simulink model "nmpcSim"  (R2024b)
settings: Solver=FixedStepAuto  StartTime=0.0  StopTime=150  RelTol=1e-3
values from neighbouring files (symbols this model uses):
  C = zeros(4,6)    [outputFcnJacobian.m]
undefined symbols (not defined in the file or in its folder): A, B, Dx, Dy, p_msg, R_gps, R_imu, R_mag, Ts, Ts_gps, Ts_imu, Ts_mag, wps, x_ref, x_ref2, y_ref, y_ref2
libraries: simulink x4, sharedTrackingLibrary x1, dspstat3 x1, mpclib x1
settings Model: Creator=mpilo  LastModifiedBy=mpilo

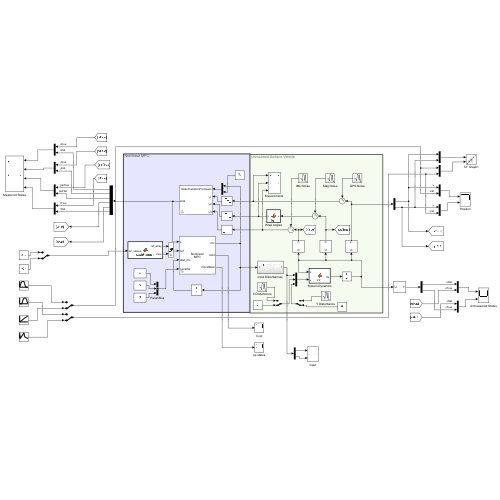
[thumbnail: Simulink's stored preview of the top-level diagram]
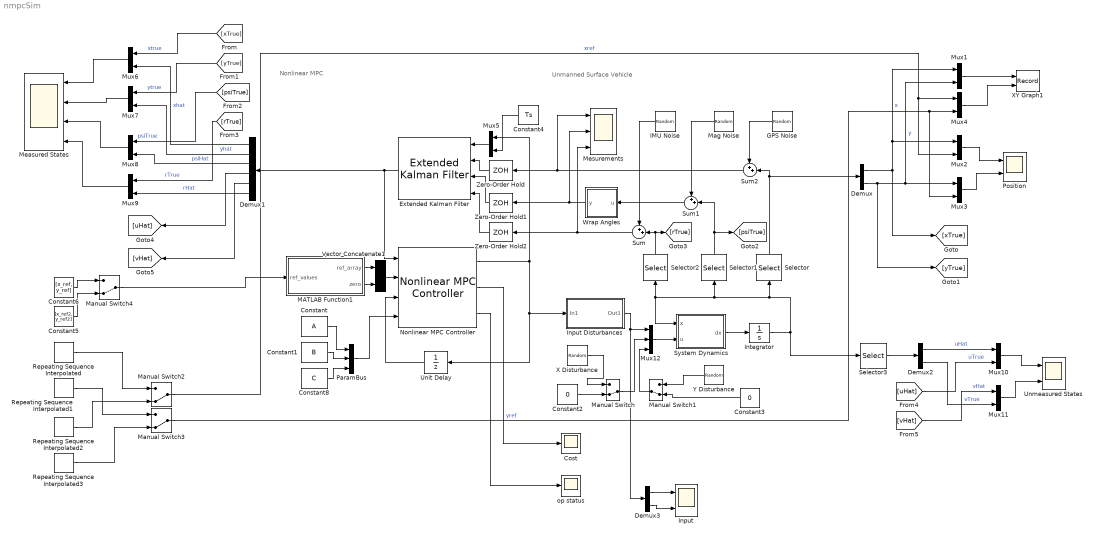
== system nmpcSim ==
  note: Nonlinear MPC
  note: Unmanned Surface Vehicle
  Constant : Constant  Value=A
  Constant1 : Constant  Value=B
  Constant2 : Constant  Value=0
  Constant3 : Constant  Value=0
  Constant4 : Constant  Value=Ts
  Constant5 : Constant  Value=[x_ref2, y_ref2]
  Constant6 : Constant  Value=[x_ref, y_ref]
  Constant8 : Constant  Value=C
  Cost : Scope
  Demux : Demux  Outputs=2
  Demux1 : Demux  Outputs=6
  Demux2 : Demux  Outputs=2
  Demux3 : Demux  Outputs=2
  Extended Kalman Filter : sharedTrackingLibrary/Extended Kalman Filter  StateTransitionFcn=stateTransitionFcnDT  HasStateTransitionJacobianFcn=off  StateTransitionJacobianFcn=stateTransitionFcnJacobian  HasAdditiveProcessNoise=Additive  ProcessNoise=Q  HasTimeVaryingProcessNoise=off  HasStateTransitionFcnExtraArgument=1  InitialState=x0  InitialStateCovariance=P_0  MeasurementFcn1=gpsMeasurementFcn  HasMeasurementJacobianFcn1=off  HasMeasurementEnablePort1=off  HasAdditiveMeasurementNoise1=Additive  MeasurementNoise1=R_gps  HasTimeVaryingMeasurementNoise1=off  HasMeasurementFcnExtraArgument1=0  HasMeasurementWrapping1=off  MeasurementFcn2=magMeasurementFcn  HasMeasurementJacobianFcn2=off  HasMeasurementEnablePort2=off  HasAdditiveMeasurementNoise2=Additive  MeasurementNoise2=R_mag  HasTimeVaryingMeasurementNoise2=off  HasMeasurementFcnExtraArgument2=0  HasMeasurementWrapping2=on  MeasurementFcn3=imuMeasurementFcn  HasMeasurementJacobianFcn3=off  HasMeasurementEnablePort3=off  HasAdditiveMeasurementNoise3=Additive  MeasurementNoise3=R_imu  HasTimeVaryingMeasurementNoise3=off  HasMeasurementFcnExtraArgument3=0  HasMeasurementWrapping3=off  MeasurementFcn4=myMeasurementFcn  HasMeasurementJacobianFcn4=off  HasMeasurementEnablePort4=off  HasAdditiveMeasurementNoise4=Additive  MeasurementNoise4=1  HasTimeVaryingMeasurementNoise4=off  HasMeasurementFcnExtraArgument4=0  HasMeasurementWrapping4=off  MeasurementFcn5=myMeasurementFcn  HasMeasurementJacobianFcn5=off  HasMeasurementEnablePort5=off  HasAdditiveMeasurementNoise5=Additive  MeasurementNoise5=1  HasTimeVaryingMeasurementNoise5=off  HasMeasurementFcnExtraArgument5=0  HasMeasurementWrapping5=off  EnableMultirate=on  StateTransitionFcnSampleTime=Ts  MeasurementFcn1SampleTime=Ts_gps  MeasurementFcn2SampleTime=Ts_mag  MeasurementFcn3SampleTime=Ts  MeasurementFcn4SampleTime=1  MeasurementFcn5SampleTime=1  UseCurrentEstimator=on  OutputStateCovariance=off  DataType=double  SampleTime=1  NumberOfMeasurements=3
      settings: LibrarySourceBlock=slident/Estimators/Extended Kalman Filter
  GPS Noise : RandomNumber  Variance=[R_gps(1,1);R_gps(2,2)]  SampleTime=Ts_gps
  IMU Noise : RandomNumber  Variance=R_imu  SampleTime=Ts_imu
  Input : Scope  NumInputPorts=2
  "Input Disturbances " : Subsystem
  Integrator : Integrator  InitialCondition=[0;0;0;0;0;0]
  MATLAB Function1 : MATLAB Function  TreatAsAtomicUnit=on
  Mag Noise : RandomNumber  Variance=R_mag  SampleTime=Ts_mag
  Manual Switch{,1..3} (4 alike) : ManualSwitch  CurrentSetting=0
  Manual Switch4 : ManualSwitch  CurrentSetting=0  varsize=on
  Measured States : Scope  NumInputPorts=4
  Mesurements : Scope  NumInputPorts=3
  Mux{1..11} (11 alike) : Mux  Inputs=2
  Mux12 : Mux  Inputs=3
  Nonlinear MPC Controller : mpclib/Nonlinear MPC Controller  nlmpcobj=nlobj  UseObjectTs=on  UseMEX=off  mexname=nmpcController  md_enabled=off  mvtarget_enabled=off  param_enabled=on  cost_enabled=on  mvseq_enabled=off  stateseq_enabled=off  ovseq_enabled=off  slack_enabled=off  status_enabled=on  ov_min=off  ov_max=off  mv_min=off  mv_max=off  mvrate_min=off  mvrate_max=off  state_min=off  state_max=off  ov_weight=off  mv_weight=off  mvrate_weight=off  ecr_weight=off  nlp_initialize=off
  ParamBus : BusCreator  Inputs=3  OutDataTypeStr=Bus: ParamBus  NonVirtualBus=on
      settings: InheritFromInputs=off
  Position : Scope  NumInputPorts=2
  Repeating Sequence Interpolated : simulink/Sources/Repeating Sequence Interpolated  OutValues=wps(:,1)  TimeValues=toa  LookUpMeth=Interpolation-Use End Values  tsamp=Ts  OutMin=[]  OutMax=[]  OutDataTypeStr=double  OutputDataTypeScalingMode=double  OutDataType=fixdt(0,8)  OutScaling=2^-10
  Repeating Sequence Interpolated1 : simulink/Sources/Repeating Sequence Interpolated  OutValues=wps(:,2)  TimeValues=toa  LookUpMeth=Interpolation-Use End Values  tsamp=Ts  OutMin=[]  OutMax=[]  OutDataTypeStr=double  OutputDataTypeScalingMode=double  OutDataType=fixdt(0,8)  OutScaling=2^-10
  Repeating Sequence Interpolated2 : simulink/Sources/Repeating Sequence Interpolated  OutValues=wps2  TimeValues=toa2  LookUpMeth=Interpolation-Use End Values  tsamp=Ts  OutMin=[]  OutMax=[]  OutDataTypeStr=double  OutputDataTypeScalingMode=double  OutDataType=fixdt(0,8)  OutScaling=2^-10
  Repeating Sequence Interpolated3 : simulink/Sources/Repeating Sequence Interpolated  OutValues=wps3  TimeValues=toa3  LookUpMeth=Interpolation-Use End Values  tsamp=Ts  OutMin=[]  OutMax=[]  OutDataTypeStr=double  OutputDataTypeScalingMode=double  OutDataType=fixdt(0,8)  OutScaling=2^-10
  Selector : Selector  InputPortWidth=6  IndexOptions=Index vector (dialog)  Indices=[1 2]  OutputSizes=1
  Selector1 : Selector  InputPortWidth=6  IndexOptions=Index vector (dialog)  Indices=3  OutputSizes=1
  Selector2 : Selector  InputPortWidth=6  IndexOptions=Index vector (dialog)  Indices=6  OutputSizes=1
  Selector3 : Selector  InputPortWidth=6  IndexOptions=Index vector (dialog)  Indices=[4 5]  OutputSizes=1
  Sum : Sum  Inputs=++|
  Sum1 : Sum  Inputs=++|
  Sum2 : Sum  Inputs=++|
  System Dynamics : MATLAB Function  TreatAsAtomicUnit=on
  Unit Delay : UnitDelay  InitialCondition=[0;0]  SampleTime=Ts  HasFrameUpgradeWarning=on
  Unmeasured States : Scope  NumInputPorts=2
  Vector Concatenate1 : Concatenate  Mode=Multidimensional array  ConcatenateDimension=2
  Wrap Angles : MATLAB Function  TreatAsAtomicUnit=on
  X Disturbance : RandomNumber  Mean=Dx.mu  Variance=Dx.sigma^2  SampleTime=Ts_imu
  XY Graph1 : Record  FileSettingsInternal="{\"entries\":[{\"content\":{\"excelSettings\":{\"content\":{},\"type\":\"Streamout.ExcelSettings\"}},\"type\":\"Streamout.FileSettingStorage\",\"uuid\":\"\"}],\"packageUris\":[\"http:\\/\\/schema.mathworks.com\\/mf0\\/streamout_blocks\\/R2020a\"],\"version\":\"1.0\"}"  Layout=[1 1]  SignalsInternal="{\"entries\":[{\"content\":{\"signals\":[{\"content\":{\"blockPath\":[],\"dimensions\":[2],\"domain\":\"\",\"hasChildren\":true,\"lineColor\":\"#77ac30\",\"lineWidth\":2,\"port\":1,\"signalID\":1,\"signalName\":\"Mux1\"},\"type\":\"RecordBlkView.Signal\",\"uuid\":\"\"},{\"content\":{\"blockPath\":[],\"channel\":[1],\"dimensions\":[2],\"domain\":\"\",\"lineColor\":\"#7e2f8e\",\"lineWidth\":2,\"parentID\":1,\"plots\":[ 1 ],\"port\":1,\"signalID\":2,\"signalName\":\"Mux1\"},\"type\":\"RecordBlkView.Signal\",\"uuid\":\"\"},{\"content\":{\"blockPath\":[],\"channel\":[2],\"dimensions\":[2],\"domain\":\"\",\"lineColor\":\"#ff6929\",\"lineWidth\":2,\"parentID\":1,\"plots\":[ 1 ],\"port\":1,\"signalID\":3,\"signalName\":\"Mux1\"},\"type\":\"RecordBlkView.Signal\",\"uuid\":\"\"},{\"content\":{\"blockPath\":[],\"dimensions\":[2],\"domain\":\"\",\"hasChildren\":true,\"lineColor\":\"#a2142f\",\"lineWidth\":2,\"port\":2,\"signalID\":4,\"signalName\":\"Mux4\"},\"type\":\"RecordBlkView.Signal\",\"uuid\":\"\"},{\"content\":{\"blockPath\":[],\"channel\":[1],\"dimensions\":[2],\"domain\":\"\",\"lineColor\":\"#4dbeee\",\"lineWidth\":2,\"parentID\":4,\"plots\":[ 1 ],\"port\":2,\"signalID\":5,\"signalName\":\"Mux4\"},\"type\":\"RecordBlkView.Signal\",\"uuid\":\"\"},{\"content\":{\"blockPath\":[],\"channel\":[2],\"dimensions\":[2],\"domain\":\"\",\"lineColor\":\"#b746ff\",\"lineWidth\":2,\"parentID\":4,\"plots\":[ 1 ],\"port\":2,\"signalID\":6,\"signalName\":\"Mux4\"},\"type\":\"RecordBlkView.Signal\",\"uuid\":\"\"}]},\"type\":\"RecordBlkView.InputSignals\",\"uuid\":\"\"}],\"packageUris\":[\"http:\\/\\/schema.mathworks.com\\/mf0\\/streamout_blocks\\/R2020a\"],\"version\":\"1.0\"}"  VisualizationBindings="{\"xyplotplugin\":{\"info\":[{\"series\":[{\"bindingParametersList\":[{\"parameter\":\"X-Axis\",\"signalID\":3,\"signalName\":\"Mux1(2)\"},{\"parameter\":\"Y-Axis\",\"signalID\":2,\"signalName\":\"Mux1(1)\"}],\"seriesID\":0},{\"bindingParametersList\":[{\"parameter\":\"X-Axis\",\"signalID\":6,\"signalName\":\"Mux4(2)\"},{\"parameter\":\"Y-Axis\",\"signalID\":5,\"signalName\":\"Mux4(1)\"}],\"seriesID\":1}],\"subplotID\":1}]}}"  CompatibilityTag=XY
  Y Disturbance : RandomNumber  Mean=Dy.mu  Variance=Dy.sigma^2  SampleTime=Ts_imu
  Zero-Order Hold : ZeroOrderHold  SampleTime=Ts_gps
  Zero-Order Hold1 : ZeroOrderHold  SampleTime=Ts_mag
  Zero-Order Hold2 : ZeroOrderHold  SampleTime=Ts
  op status : Scope
  wires:
  Manual Switch2/1 -> Mux2/2, Mux4/1  "xref"
  Mux3/1 -> Position/2
  Integrator/1 -> Selector3/1, Selector1/1, Selector2/1, System Dynamics/1(x), Selector/1
  Demux/2 -> [yTrue], Mux1/2, Mux3/1  "y"
  Unit Delay/1 -> Nonlinear MPC Controller/3
  Demux3/1 -> Input/1
  Demux3/2 -> Input/2
  Demux/1 -> Mux2/1, Mux1/1, [xTrue]  "x"
  Manual Switch3/1 -> Mux3/2, Mux4/2  "yref"
  Vector Concatenate1/1 -> Nonlinear MPC Controller/2
  Mux2/1 -> Position/1
  System Dynamics/1(dx) -> Integrator/1
  Mux1/1 -> XY Graph1/1
  Mux4/1 -> XY Graph1/2
  Nonlinear MPC Controller/2 -> Cost/1
  Repeating Sequence Interpolated/1 -> Manual Switch2/1
  Repeating Sequence Interpolated2/1 -> Manual Switch2/2
  Repeating Sequence Interpolated1/1 -> Manual Switch3/1
  Repeating Sequence Interpolated3/1 -> Manual Switch3/2
  Constant/1 -> ParamBus/1
  ParamBus/1 -> Nonlinear MPC Controller/4
  Constant1/1 -> ParamBus/2
  Extended Kalman Filter/1 -> Demux1/1, Nonlinear MPC Controller/1
  Selector2/1 -> [rTrue], Sum/2
  Selector1/1 -> Sum1/2, [psiTrue]
  IMU Noise/1 -> Sum/1
  Mag Noise/1 -> Sum1/1
  Sum/1 -> Mesurements/3, Zero-Order Hold2/1
  Sum1/1 -> Wrap Angles/1(u)
  Sum2/1 -> Mesurements/1, Zero-Order Hold/1
  Mux5/1 -> Extended Kalman Filter/1
  Constant4/1 -> Mux5/2
  Nonlinear MPC Controller/1 -> "Input Disturbances "/1(In1), Unit Delay/1, Mux5/1
  [yTrue] -> Mux7/1  "ytrue"
  Demux1/3 -> Mux8/2  "psiHat"
  Demux1/4 -> [uHat]
  Mux7/1 -> Measured States/2
  [psiTrue] -> Mux8/1  "psiTrue"
  Demux1/2 -> Mux7/2  "yhat"
  Mux8/1 -> Measured States/3
  Demux1/1 -> Mux6/2  "xhat"
  [xTrue] -> Mux6/1  "xtrue"
  Mux6/1 -> Measured States/1
  Demux1/5 -> [vHat]
  Mux9/1 -> Measured States/4
  [rTrue] -> Mux9/1  "rTrue"
  Demux1/6 -> Mux9/2  "rHat"
  Zero-Order Hold2/1 -> Extended Kalman Filter/4
  Mux10/1 -> Unmeasured States/1
  Mux11/1 -> Unmeasured States/2
  Selector3/1 -> Demux2/1
  Demux2/1 -> Mux10/1  "uHat"
  Demux2/2 -> Mux11/2  "vTrue"
  [uHat] -> Mux10/2  "uTrue"
  [vHat] -> Mux11/1  "vHat"
  Zero-Order Hold/1 -> Extended Kalman Filter/2
  Zero-Order Hold1/1 -> Extended Kalman Filter/3
  Wrap Angles/1(y) -> Mesurements/2, Zero-Order Hold1/1
  GPS Noise/1 -> Sum2/1
  X Disturbance/1 -> Manual Switch/1
  Y Disturbance/1 -> Manual Switch1/1
  Mux12/1 -> System Dynamics/2(u)
  Manual Switch/1 -> Mux12/2
  Manual Switch1/1 -> Mux12/3
  Constant2/1 -> Manual Switch/2
  Constant3/1 -> Manual Switch1/2
  Constant8/1 -> ParamBus/3
  Nonlinear MPC Controller/3 -> op status/1
  "Input Disturbances "/1(Out1) -> Mux12/1, Demux3/1
  Selector/1 -> Sum2/2, Demux/1
  Constant6/1 -> Manual Switch4/1
  Manual Switch4/1 -> MATLAB Function1/1(ref_values)
  Constant5/1 -> Manual Switch4/2
  MATLAB Function1/2(zero) -> Vector Concatenate1/2
  MATLAB Function1/1(ref_array) -> Vector Concatenate1/1

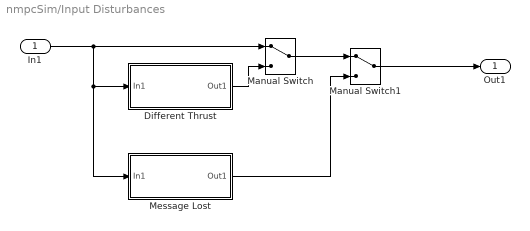
== system nmpcSim/Input Disturbances  ==
  In1 : Inport
  Different Thrust : Subsystem
  Manual Switch : ManualSwitch
  Manual Switch1 : ManualSwitch
  Message Lost : Subsystem
  Out1 : Outport
  wires:
  In1/1 -> Manual Switch/1, Message Lost/1(In1), Different Thrust/1(In1)
  Manual Switch/1 -> Manual Switch1/1
  Manual Switch1/1 -> Out1/1
  Different Thrust/1(Out1) -> Manual Switch/2
  Message Lost/1(Out1) -> Manual Switch1/2

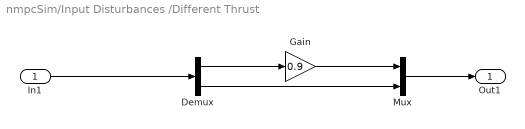
== system nmpcSim/Input Disturbances /Different Thrust ==
  In1 : Inport
  Demux : Demux  Outputs=2
  Gain : Gain  Gain=0.9
  Mux : Mux  Inputs=2
  Out1 : Outport
  wires:
  In1/1 -> Demux/1
  Demux/1 -> Gain/1
  Gain/1 -> Mux/1
  Demux/2 -> Mux/2
  Mux/1 -> Out1/1

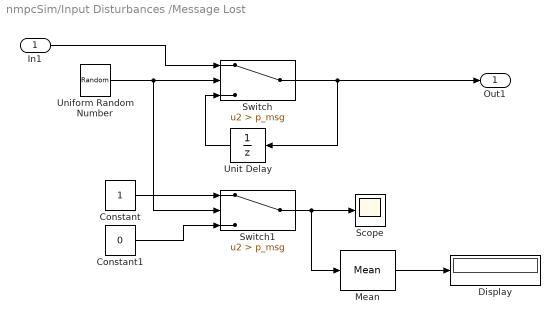
== system nmpcSim/Input Disturbances /Message Lost ==
  In1 : Inport
  Constant : Constant
  Constant1 : Constant  Value=0
  Display : Display
  Mean : dspstat3/Mean  run=on  reset_popup=None  directionMode=Each column  dimension=1  roiEnable=off  roiType=Rectangles  roiPortion=Entire ROI  roiOutput=Individual statistics for each ROI  roiFlag=off  roundingMode=Floor  overflowMode=off  outputDataTypeStr=Inherit: Same as accumulator  outputMin=[]  outputMax=[]  outputLastDataTypeStr=Inherit: Same as accumulator
  Scope : Scope
  Switch : Switch  Criteria=u2 > Threshold  Threshold=p_msg  SaturateOnIntegerOverflow=off  InputSameDT=off
  Switch1 : Switch  Criteria=u2 > Threshold  Threshold=p_msg  SaturateOnIntegerOverflow=off  InputSameDT=off
  Uniform Random Number : UniformRandomNumber  Minimum=0  SampleTime=Ts
  Unit Delay : UnitDelay  SampleTime=Ts  HasFrameUpgradeWarning=on
  Out1 : Outport
  wires:
  Switch/1 -> Unit Delay/1, Out1/1
  In1/1 -> Switch/1
  Uniform Random Number/1 -> Switch1/2, Switch/2
  Unit Delay/1 -> Switch/3
  Constant/1 -> Switch1/1
  Constant1/1 -> Switch1/3
  Switch1/1 -> Mean/1, Scope/1
  Mean/1 -> Display/1

== matlab function nmpcSim/Wrap Angles ==
  data: u input; y output
function y = fcn(u)
% Heading is bounded between 0 and 360 degrees
y = wrapTo2Pi(u);

== matlab function nmpcSim/System Dynamics ==
  data: x input; u input; dx output
function dx = SS(x, u)
%% State Space Model

% Determine state derivatives from state space equation
dx = stateTransitionFcn(x,u);
end

== matlab function nmpcSim/MATLAB Function1 ==
  data: ref_values input; ref_array output; zero output
function [ref_array, zero] = pathPlanner(ref_values)
%% Sets Reference values for NMPC controller
% ref_values: Matrix of reference values with two columns [x, y]

% Current timestep
persistent k 
if isempty(k)
    k = 1;
end

% p: Number of future values to output (including the current value)
% i.e. Predicition horizon
p = 20;

% Get the number of rows (samples) in the reference array
N = size(ref_values, 1);

% Initialise the output array (p rows for p future values, 
% 2 columns for x and y)
ref_array = zeros(p, 2);
zero = ref_array;  % Output a zero matrix of the same size for psi and r

% Loop through and fill the array with current and next p-1 values
for i = 0:(p-1)
    % Calculate the index for current value and next p-1 values
    % Using modulo operation to loop back around
    idx = mod(k + i - 1, N) + 1;
    
    % Assign [x, y] values at index idx
    ref_array(i+1, :) = ref_values(idx, :); 
end

% Increment the timestep
k = k + 1;
end
